simulink model "simulink_cruise_control_system"  (R2023b)
settings: Solver=VariableStepAuto  StartTime=0.0  StopTime=160  RelTol=1e-3
values from neighbouring files (symbols this model uses):
  A = 2.2    [cruise_control_init.m]
  Cd = 0.3    [cruise_control_init.m]
  F_engine_max = 5000    [cruise_control_init.m]
  F_engine_min = 0    [cruise_control_init.m]
  F_hill = m * g * sin(theta)    [cruise_control_init.m]
  F_roll = Crr * m * g    (= 220.725)    [cruise_control_init.m]
  Kd = 100    [cruise_control_init.m]
  Ki = 50    [cruise_control_init.m]
  Kp = 500    [cruise_control_init.m]
  m = 1500    [cruise_control_init.m]    (also in cruise_control_plots.m)
  rho = 1.225    [cruise_control_init.m]
  T_hill = 10    [cruise_control_init.m]    (also in cruise_control_plots.m = 80)
  v_target = v_target_mph * 0.44704    (= 31.2928)    [cruise_control_init.m]    (also in cruise_control_plots.m = 31.3)
libraries: slpidlib x1
settings Model: Creator=kylew  LastModifiedBy=kylew

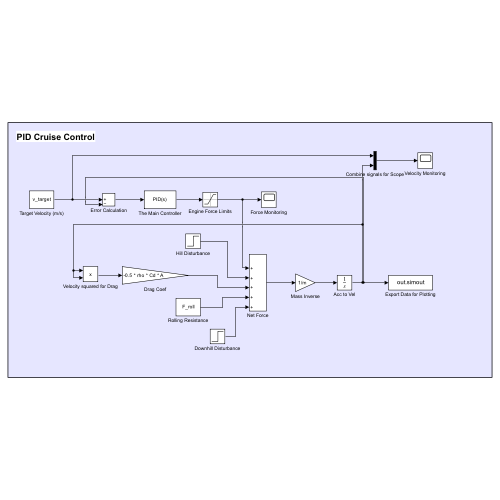
[thumbnail: Simulink's stored preview of the top-level diagram]
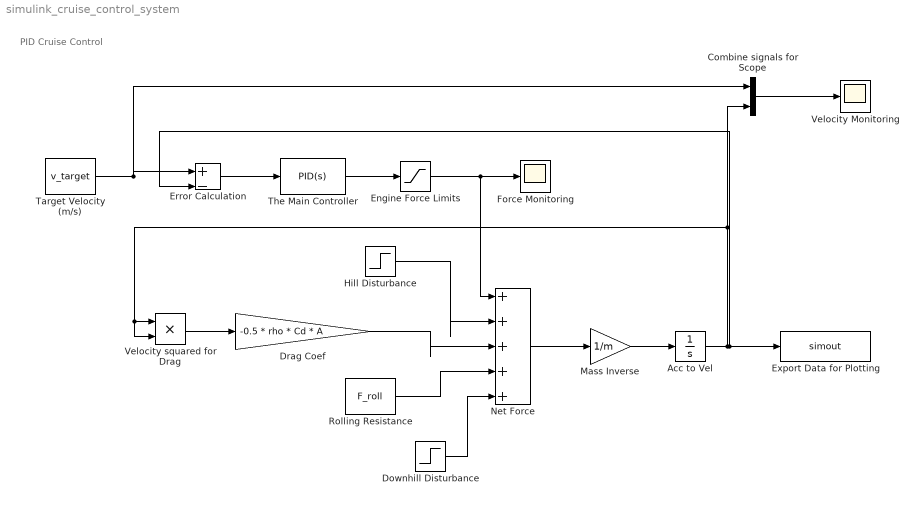
== system simulink_cruise_control_system ==
  note: PID Cruise Control
  Acc to Vel : Integrator
  Combine signals for Scope : Mux  Inputs=2
  Downhill Disturbance : Step  Time=20  After=-F_hill  SampleTime=0
  Drag Coef : Gain  Gain=-0.5 * rho * Cd * A
  Engine Force Limits : Saturate  UpperLimit=F_engine_max  LowerLimit=F_engine_min
  Error Calculation : Sum  Inputs=|+-
  Export Data for Plotting : ToWorkspace  VariableName=simout  SaveFormat=Timeseries  SampleTime=-1
  Force Monitoring : Scope
  Hill Disturbance : Step  Time=T_hill  After=F_hill  SampleTime=0
  Mass Inverse : Gain  Gain=1/m
  Net Force : Sum  Inputs=|+++++
  Rolling Resistance : Constant  Value=F_roll
  Target Velocity (m/s) : Constant  Value=v_target
  The Main Controller : slpidlib/PID Controller  Controller=PID  Form=Parallel  TimeDomain=Continuous-time  UseExternalTs=off  SampleTime=-1  IntegratorMethod=Forward Euler  FilterMethod=Forward Euler  ControllerParametersSource=internal  P=Kp  I=Ki  UseKiTs=off  D=Kd  N=100  UseFilter=on  TunerSelectOption=Transfer Function Based (PID Tuner App)  InitialConditionSource=internal  InitialConditionForIntegrator=0  InitialConditionForFilter=0  DifferentiatorICPrevScaledInput=0  ExternalReset=none  TrackingMode=off  Kt=1  LimitOutput=off  SatLimitsSource=internal  UpperSaturationLimit=inf  LowerSaturationLimit=-inf  LinearizeAsGain=on  AntiWindupMode=none  Kb=1  LimitIntegrator=off  UpperIntegratorSaturationLimit=inf  LowerIntegratorSaturationLimit=-inf  POutMin=[]  POutMax=[]  IOutMin=[]  IOutMax=[]  DOutMin=[]  DOutMax=[]  NOutMin=[]  NOutMax=[]  SumOutMin=[]  SumOutMax=[]  SaturationOutMin=[]  SaturationOutMax=[]  PParamMin=[]  PParamMax=[]  IParamMin=[]  IParamMax=[]  DParamMin=[]  DParamMax=[]  NParamMin=[]  NParamMax=[]  KbParamMin=[]  KbParamMax=[]  KtParamMin=[]  KtParamMax=[]  KbOutMin=[]  KbOutMax=[]  KtOutMin=[]  KtOutMax=[]  IntegratorOutMin=[]  IntegratorOutMax=[]  FilterOutMin=[]  FilterOutMax=[]  SumI1OutMin=[]  SumI1OutMax=[]  SumI2OutMin=[]  SumI2OutMax=[]  SumI3OutMin=[]  SumI3OutMax=[]  SumI4OutMin=[]  SumI4OutMax=[]  SumDOutMin=[]  SumDOutMax=[]  DifferentiatorOutMin=[]  DifferentiatorOutMax=[]  FilterDiffOutCoefMin=[]  FilterDiffOutCoefMax=[]  ReciprocalOutMin=[]  ReciprocalOutMax=[]  SumDenOutMin=[]  SumDenOutMax=[]  SumNumOutMin=[]  SumNumOutMax=[]  DivideOutMin=[]  DivideOutMax=[]  UdiffTsProdOutMin=[]  UdiffTsProdOutMax=[]  NTsProdOutMin=[]  NTsProdOutMax=[]  UintegralTsProdOutMin=[]  UintegralTsProdOutMax=[]  UngainTsProdOutMin=[]  UngainTsProdOutMax=[]  ClampingZeroOutDataTypeStr=Inherit: Inherit via back propagation  ClampingZeroOutMin=[]  ClampingZeroOutMax=[]  FilterDenConstantOutDataTypeStr=Inherit: Inherit via back propagation  FilterDenConstantOutMin=[]  FilterDenConstantOutMax=[]  PCopyOutDataTypeStr=Inherit: Inherit via back propagation  PCopyOutMin=[]  PCopyOutMax=[]  NCopyOutDataTypeStr=Inherit: Inherit via back propagation  NCopyOutMin=[]  NCopyOutMax=[]  IntegratorContinuousStateAttributes=''  IntegratorStateMustResolveToSignalObject=off  IntegratorRTWStateStorageClass=Auto  FilterContinuousStateAttributes=''  FilterStateMustResolveToSignalObject=off  FilterRTWStateStorageClass=Auto  ParallelPVariant=InternalParameters  IdealPVariant=Disabled  IVariant=InternalParameters  DVariant=InternalParameters  IntegratorVariant=Continuous  SatVariant=Disabled  AWVariant=Passthrough  PCopyVariant=Disabled  TRVariant=Disabled  FdbkBlocksVariant=Forward  IdealPFdbkVariant=Disabled  SatFdbkVariant=Disabled  DerivativeFilterVariant=ContFilter  NVariant=InternalParameters  NCopyVariant=Disabled  FilterICVariant=InternalICsFilter  IntegratorICVariant=InternalICs  ExternalResetVariant=Disabled  TRSumVariant=Passthrough  SumFdbkVariant=Disabled  SumVariant=Sum_PID  TsampFilterVariant=InternalTs  TsampNgainVariant=Passthrough  TsampIntegralVariant=Disabled_SignalSpec  ExternalSaturationOutDataTypeStr=Inherit: Same as second input
  Velocity Monitoring : Scope
  Velocity squared for Drag : Product
  wires:
  Error Calculation/1 -> The Main Controller/1
  Target Velocity (m/s)/1 -> Combine signals for Scope/1, Error Calculation/1
  Combine signals for Scope/1 -> Velocity Monitoring/1
  The Main Controller/1 -> Engine Force Limits/1
  Rolling Resistance/1 -> Net Force/4
  Net Force/1 -> Mass Inverse/1
  Mass Inverse/1 -> Acc to Vel/1
  Acc to Vel/1 -> Export Data for Plotting/1, Error Calculation/2, Combine signals for Scope/2, Velocity squared for Drag/2, Velocity squared for Drag/1
  Engine Force Limits/1 -> Net Force/1, Force Monitoring/1
  Hill Disturbance/1 -> Net Force/2
  Drag Coef/1 -> Net Force/3
  Velocity squared for Drag/1 -> Drag Coef/1
  Downhill Disturbance/1 -> Net Force/5
